simulink model "heat_exchanger_lab"  (R2017b)
settings: Solver=VariableStepAuto  StartTime=0.0  StopTime=10.0  RelTol=1e-3
values from neighbouring files (symbols this model uses):
  A = subs(A,var_list,var_val)    [linearization.m]
  B = [(cp_wort*(T_wort_in - x_wort_0))/(m_wort*cp_wort) 0 ... (first row only)    [heat_exchanger_config.m]    (also in linearization.m = subs(B,var_list,var_val))
  C = [1 0 ; 0 1]    [heat_exchanger_config.m]
  cp_wort = 4062    [heat_exchanger_config.m]    (also in linearization.m = 4000)
  D = zeros(length(C_exact(:,1)),length(B_exact(1,:)))    [heat_exchanger_config.m]
  Reference = [20 70]    [heat_exchanger_config.m]    (also in linearization.m = [25 16])
  rho_wort = 1.06    [heat_exchanger_config.m]    (also in linearization.m)
  x_H2O_0 = 0    [heat_exchanger_config.m]
  x_wort_0 = 0    [heat_exchanger_config.m]
undefined symbols (not defined in the file or in its folder): LQR_gain
settings Model: Creator=Alexander  LastModifiedBy=Alexander

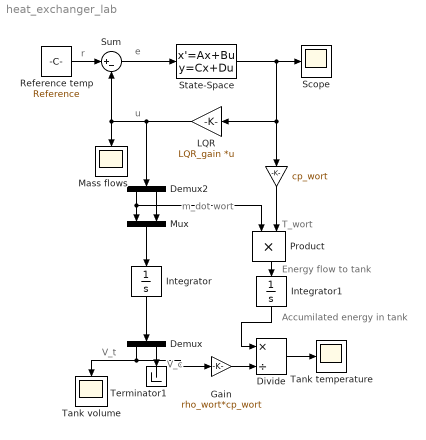
== system heat_exchanger_lab ==
  note: r
  note: V_t
  note: m_dot wort
  note: T_wort
  note: e
  note: Energy flow to tank
  note: V_c
  note: Accumilated energy in tank
  note: u
  " " : Gain  Gain=cp_wort
  Demux : Demux  Outputs=2
  Demux2 : Demux  Outputs=2
  Divide : Product  Inputs=*/
  Gain : Gain  Gain=rho_wort*cp_wort
  Integrator : Integrator
  Integrator1 : Integrator
  LQR : Gain  Gain=LQR_gain  Multiplication=Matrix(K*u) (u vector)
  Mass flows : Scope
  Mux : Mux  Inputs=2
  Product : Product
  Reference temp : Constant  Value=Reference
  Scope : Scope
  State-Space : StateSpace  A=A  B=B  C=C  D=D  InitialCondition=[x_wort_0 ; x_H2O_0]
  Sum : Sum  Inputs=|+-
  Tank temperature : Scope
  Tank volume : Scope
  Terminator1 : Terminator
  wires:
  Demux/2 -> Terminator1/1
  Integrator/1 -> Demux/1
  State-Space/1 -> Scope/1, LQR/1, " "/1
  LQR/1 -> Demux2/1, Sum/2, Mass flows/1
  Reference temp/1 -> Sum/1
  Demux2/2 -> Mux/2
  Demux2/1 -> Product/1, Mux/1
  Mux/1 -> Integrator/1
  Demux/1 -> Tank volume/1, Gain/1
  Product/1 -> Integrator1/1
  Integrator1/1 -> Divide/1
  Sum/1 -> State-Space/1
  " "/1 -> Product/2
  Divide/1 -> Tank temperature/1
  Gain/1 -> Divide/2
